simulink model "simulinkComparison"  (R2015a)
settings: Solver=ode45  StartTime=0.0  StopTime=10.0  RelTol=1e-3
settings Model: Creator=theVenom  LastModifiedBy=theVenom

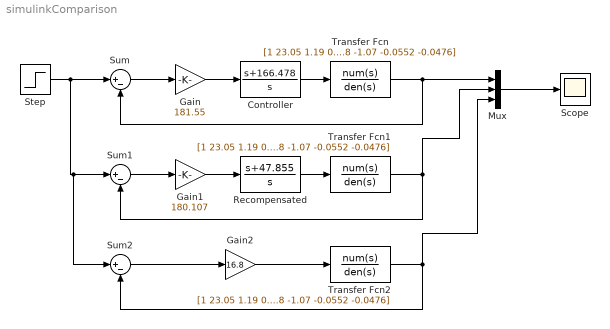
== system simulinkComparison ==
  Controller : TransferFcn  Numerator=[1 166.478]  Denominator=[1 0]
  Gain : Gain  Gain=181.55
  Gain1 : Gain  Gain=180.107
  Gain2 : Gain  Gain=16.8
  Mux : Mux  Inputs=3
  Recompensated : TransferFcn  Numerator=[1 47.855]  Denominator=[1 0]
  Scope : Scope
      settings: YMin=0.87821  YMax=1.4382
  Step : Step  SampleTime=0
  Sum : Sum  Inputs=|+-
  Sum1 : Sum  Inputs=|+-
  Sum2 : Sum  Inputs=|+-
  Transfer Fcn : TransferFcn  Numerator=[1 23.05 1.19 0.92]  Denominator=[1 1.08 -1.07 -0.0552 -0.0476]
  Transfer Fcn1 : TransferFcn  Numerator=[1 23.05 1.19 0.92]  Denominator=[1 1.08 -1.07 -0.0552 -0.0476]
  Transfer Fcn2 : TransferFcn  Numerator=[1 23.05 1.19 0.92]  Denominator=[1 1.08 -1.07 -0.0552 -0.0476]
  wires:
  Transfer Fcn/1 -> Mux/1, Sum/2
  Sum/1 -> Gain/1
  Gain/1 -> Controller/1
  Controller/1 -> Transfer Fcn/1
  Transfer Fcn1/1 -> Sum1/2, Mux/2
  Sum1/1 -> Gain1/1
  Gain1/1 -> Recompensated/1
  Recompensated/1 -> Transfer Fcn1/1
  Transfer Fcn2/1 -> Sum2/2, Mux/3
  Step/1 -> Sum2/1, Sum1/1, Sum/1
  Sum2/1 -> Gain2/1
  Gain2/1 -> Transfer Fcn2/1
  Mux/1 -> Scope/1
